simulink model "q3_d"  (R2026a)
settings: Solver=FixedStepDiscrete  FixedStep=0.1  EnableMultiTasking=on
model workspace (MAT data in the model file):
  e = Simulink.Parameter
  e.Value = 2
  e.Complexity = 'real'
  e.Dimensions = [1 1]
  e.DataType = 'auto'
values from neighbouring files (symbols this model uses):
  T = Simulink.Parameter    [q3_variables.m]
settings Model: Creator=LAB_PC  LastModifiedBy=LAB_PC

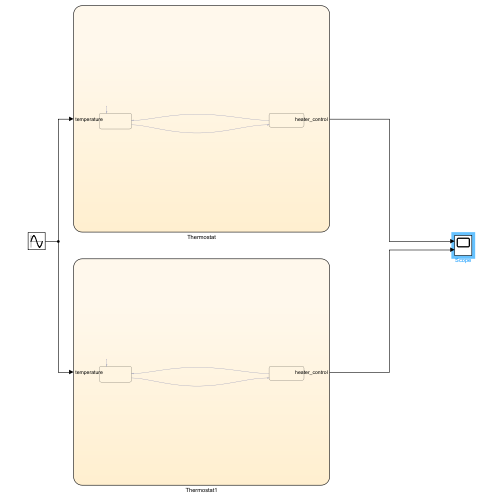
[thumbnail: Simulink's stored preview of the top-level diagram]
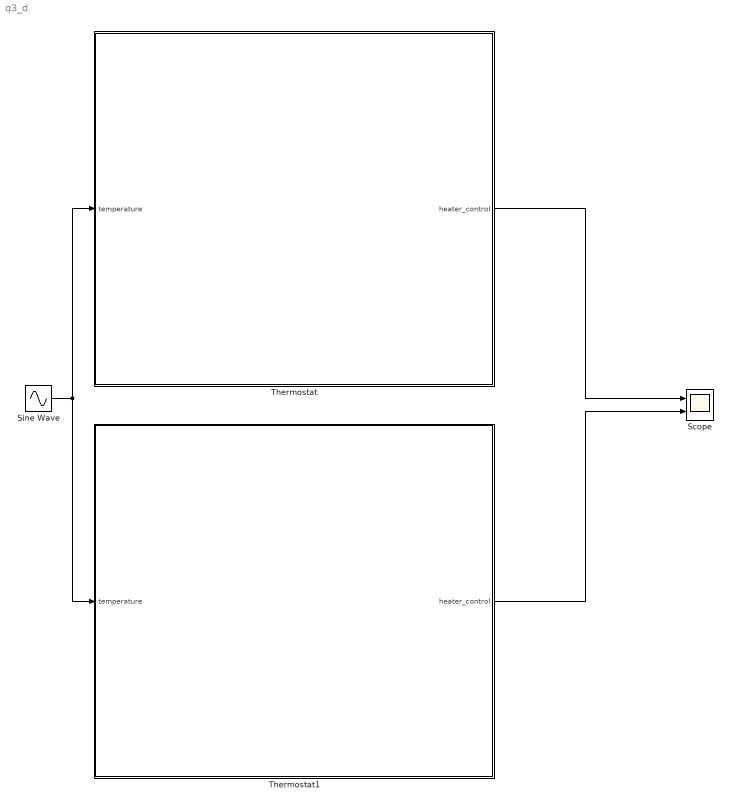
== system q3_d ==
  Scope : Scope  NumInputPorts=2
      settings: ActiveDisplayYMinimum=-5.7039603040669729  ActiveDisplayYMaximum=5.2108468566197281
  Sine Wave : Sin  Amplitude=5  Bias=24  SampleTime=0
  Thermostat : Stateflow chart  TreatAsAtomicUnit=on
  Thermostat1 : Stateflow chart  TreatAsAtomicUnit=on
  wires:
  Thermostat/1(heater_control) -> Scope/1
  Sine Wave/1 -> Thermostat/1(temperature), Thermostat1/1(temperature)
  Thermostat1/1(heater_control) -> Scope/2

== stateflow chart q3_d/Thermostat1 ==
  state Cooling
    entry:heater_control=0;
  state Heating
    entry: heater_control = 1;
  (default) -> Cooling
  Heating -> Cooling : [temperature > T+e]
  Cooling -> Heating : [temperature <T-e]
  data: heater_control output; temperature input; T parameter; e parameter

== stateflow chart q3_d/Thermostat ==
  state Cooling
    entry:heater_control=0;
  state Heating
    entry: heater_control = 1;
  (default) -> Cooling
  Heating -> Cooling : [temperature > T]
  Cooling -> Heating : [temperature <T]
  data: heater_control output; temperature input; T parameter
